simulink library "robot1"
PostLoadFcn:
  | robot1_BusGenerator
libraries: AtomicLibrary x3

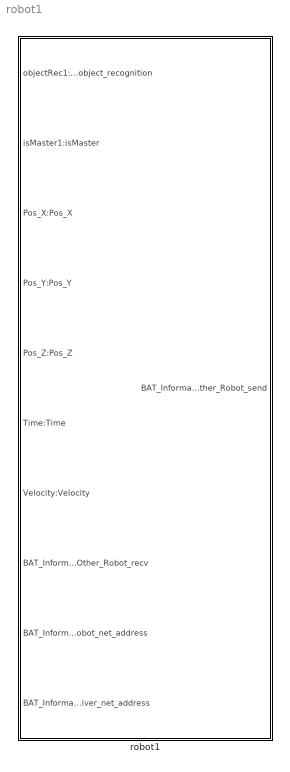
== system robot1 ==
  robot1 : Subsystem  Tag=id=_8vFAgJMGEeKkUdL0M2Clrg

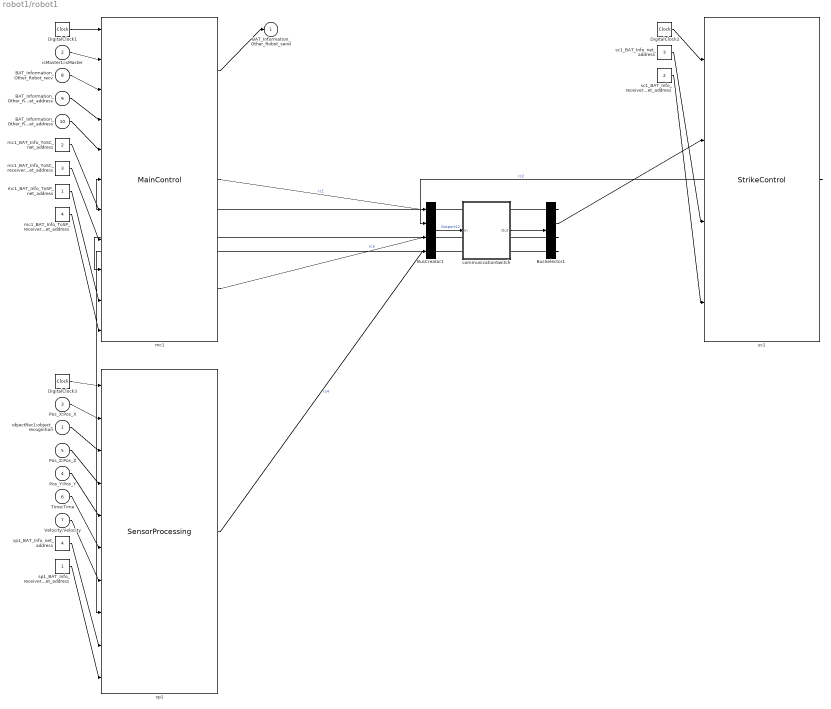
== system robot1/robot1 ==
  objectRec1:object_recognition : Inport  Tag=id=_98BUwJMGEeKkUdL0M2Clrg  Port=1  DataType=boolean  OutDataType=fixdt(1, 16)  OutScaling=2^0  OutDataTypeStr=boolean
  isMaster1:isMaster : Inport  Tag=id=_98QlUJMGEeKkUdL0M2Clrg  Port=2  DataType=boolean  OutDataType=fixdt(1, 16)  OutScaling=2^0  OutDataTypeStr=boolean
  Pos_X:Pos_X : Inport  Tag=id=_98nxsJMGEeKkUdL0M2Clrg  Port=3  DataType=boolean  OutDataType=fixdt(1, 16)  OutScaling=2^0  OutDataTypeStr=boolean
  Pos_Y:Pos_Y : Inport  Tag=id=_989v8JMGEeKkUdL0M2Clrg  Port=4  DataType=boolean  OutDataType=fixdt(1, 16)  OutScaling=2^0  OutDataTypeStr=boolean
  Pos_Z:Pos_Z : Inport  Tag=id=_99THIJMGEeKkUdL0M2Clrg  Port=5  DataType=boolean  OutDataType=fixdt(1, 16)  OutScaling=2^0  OutDataTypeStr=boolean
  Time:Time : Inport  Tag=id=_99svwJMGEeKkUdL0M2Clrg  Port=6  DataType=boolean  OutDataType=fixdt(1, 16)  OutScaling=2^0  OutDataTypeStr=boolean
  Velocity:Velocity : Inport  Tag=id=_9-QwcJMGEeKkUdL0M2Clrg  Port=7  DataType=boolean  OutDataType=fixdt(1, 16)  OutScaling=2^0  OutDataTypeStr=boolean
  BAT_Information_Other_Robot_recv : Inport  Tag=id=_9_CMgJMGEeKkUdL0M2Clrg  Port=8  DataType=auto  OutDataType=fixdt(1, 16)  OutScaling=2^0  UseBusObject=on  OutDataTypeStr=Inherit: auto
      settings: BusObject=PacketBus
  BAT_Information_Other_Robot_net_address : Inport  Tag=id=_9_CzkZMGEeKkUdL0M2Clrg  Port=9  DataType=uint8  OutDataType=fixdt(1, 16)  OutScaling=2^0  OutDataTypeStr=uint8
  BAT_Information_Other_Robot_receiver_net_address : Inport  Tag=id=_9_DaoJMGEeKkUdL0M2Clrg  Port=10  DataType=uint8  OutDataType=fixdt(1, 16)  OutScaling=2^0  OutDataTypeStr=uint8
  BAT_Information_Other_Robot_send : Outport  Tag=id=_9_CzkJMGEeKkUdL0M2Clrg  Port=1  DataType=auto  OutDataType=fixdt(1, 16)  OutScaling=2^0  UseBusObject=on  OutDataTypeStr=Inherit: auto
      settings: BusObject=PacketBus
  communicationSwitch : Subsystem  Tag=id=_8vJR8pMGEeKkUdL0M2Clrg
  BusCreator1 : BusCreator  Inputs=4  UseBusObject=on  Tag=id=_8vGOoJMGEeKkUdL0M2Clrg
      settings: BusObject=robot1_Bus
  BusSelector1 : BusSelector  OutputSignals=rc1,rc2,rc3,rc4  Tag=id=_8vGOoZMGEeKkUdL0M2Clrg
  mc1 : AtomicLibrary/MainControl  Tag=id=_8wMa0JMGEeKkUdL0M2Clrg
  DigitalClock1 : DigitalClock  Tag=id=_8wMa0ZMGEeKkUdL0M2Clrg  SampleTime=0.0010
  sc1 : AtomicLibrary/StrikeControl  Tag=id=_8wPeIZMGEeKkUdL0M2Clrg
  DigitalClock2 : DigitalClock  Tag=id=_8wQFMJMGEeKkUdL0M2Clrg  SampleTime=0.0010
  sp1 : AtomicLibrary/SensorProcessing  Tag=id=_8wShcZMGEeKkUdL0M2Clrg
  DigitalClock3 : DigitalClock  Tag=id=_8wTIgJMGEeKkUdL0M2Clrg  SampleTime=0.0010
  mc1_BAT_Info_ToSC_net_address : Constant  Tag=id=_94PA8ZMGEeKkUdL0M2Clrg  Value=2  OutDataTypeMode=uint8  OutDataTypeStr=uint8
  mc1_BAT_Info_ToSP_net_address : Constant  Tag=id=_94dDYZMGEeKkUdL0M2Clrg  Value=1  OutDataTypeMode=uint8  OutDataTypeStr=uint8
  sc1_BAT_Info_net_address : Constant  Tag=id=_94qewZMGEeKkUdL0M2Clrg  Value=3  OutDataTypeMode=uint8  OutDataTypeStr=uint8
  sp1_BAT_Info_net_address : Constant  Tag=id=_95kdsZMGEeKkUdL0M2Clrg  Value=4  OutDataTypeMode=uint8  OutDataTypeStr=uint8
  mc1_BAT_Info_ToSC_receiver_net_address : Constant  Tag=id=_GLOx5ZMHEeKkUdL0M2Clrg  Value=3  OutDataTypeMode=uint8  OutDataTypeStr=uint8
  sc1_BAT_Info_receiver_net_address : Constant  Tag=id=_GLQAAJMHEeKkUdL0M2Clrg  Value=2  OutDataTypeMode=uint8  OutDataTypeStr=uint8
  mc1_BAT_Info_ToSP_receiver_net_address : Constant  Tag=id=_GLZxBJMHEeKkUdL0M2Clrg  Value=4  OutDataTypeMode=uint8  OutDataTypeStr=uint8
  sp1_BAT_Info_receiver_net_address : Constant  Tag=id=_GLa_IZMHEeKkUdL0M2Clrg  Value=1  OutDataTypeMode=uint8  OutDataTypeStr=uint8
  wires:
  BusCreator1/1 -> communicationSwitch/1(In)  "Outport12"
  communicationSwitch/1(Out) -> BusSelector1/1
  DigitalClock1/1 -> mc1/1
  DigitalClock2/1 -> sc1/1
  DigitalClock3/1 -> sp1/1
  mc1_BAT_Info_ToSC_net_address/1 -> mc1/7
  mc1_BAT_Info_ToSP_net_address/1 -> mc1/10
  sc1_BAT_Info_net_address/1 -> sc1/3
  sp1_BAT_Info_net_address/1 -> sp1/9
  mc1/2 -> BusCreator1/1  "rc1"
  sc1/1 -> BusCreator1/2  "rc2"
  BusSelector1/2 -> sc1/2
  BusSelector1/1 -> mc1/6
  mc1_BAT_Info_ToSC_receiver_net_address/1 -> mc1/8
  sc1_BAT_Info_receiver_net_address/1 -> sc1/4
  mc1/3 -> BusCreator1/3  "rc3"
  sp1/1 -> BusCreator1/4  "rc4"
  BusSelector1/4 -> sp1/8
  BusSelector1/3 -> mc1/9
  mc1_BAT_Info_ToSP_receiver_net_address/1 -> mc1/11
  sp1_BAT_Info_receiver_net_address/1 -> sp1/10
  isMaster1:isMaster/1 -> mc1/2
  Pos_Z:Pos_Z/1 -> sp1/4
  Pos_Y:Pos_Y/1 -> sp1/5
  Pos_X:Pos_X/1 -> sp1/2
  Time:Time/1 -> sp1/6
  objectRec1:object_recognition/1 -> sp1/3
  Velocity:Velocity/1 -> sp1/7
  BAT_Information_Other_Robot_recv/1 -> mc1/3
  mc1/1 -> BAT_Information_Other_Robot_send/1
  BAT_Information_Other_Robot_receiver_net_address/1 -> mc1/5
  BAT_Information_Other_Robot_net_address/1 -> mc1/4

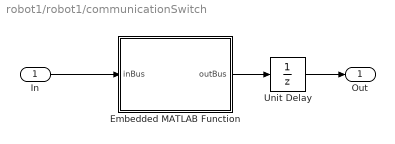
== system robot1/robot1/communicationSwitch ==
  In : Inport  Tag=id=_8vMVQJMGEeKkUdL0M2Clrg  Port=1  PortDimensions=-1  OutDataType=fixdt(1, 16)  OutScaling=2^0  UseBusObject=on
      settings: BusObject=robot1_Bus
  Out : Outport  Tag=id=_8vOKcJMGEeKkUdL0M2Clrg  Port=1  PortDimensions=-1  OutDataType=fixdt(1, 16)  OutScaling=2^0  UseBusObject=on
      settings: BusObject=robot1_Bus
  Unit Delay : UnitDelay  Tag=id=_8vPYkJMGEeKkUdL0M2Clrg  SampleTime=-1
  Embedded MATLAB Function : Stateflow chart  Tag=id=_8vPYkZMGEeKkUdL0M2Clrg
  wires:
  In/1 -> Embedded MATLAB Function/1(inBus)
  Unit Delay/1 -> Out/1
  Embedded MATLAB Function/1(outBus) -> Unit Delay/1

== matlab function robot1/communicationSwitch/Embedded MATLAB Function ==
  data: inBus input Bus: robot1_Bus; outBus output Bus: robot1_Bus
function outBus = BusImpl(inBus)
%#eml
eml.extrinsic('fieldnames','disp','setfield','fprintf');

busSize = 1;
queueSize = 10*busSize; %length of queue
numShuttles = 0; %Define data type
numShuttles = numel(fieldnames(inBus)); %Shuttles connected to the bus
assert(numShuttles <= 20) %Defines an upper bound for number of shuttles. 
%Important for static memory allocation. 
lookupTableSize = 200;



NOT_ASSIGNED = -1;

%We need persistent queues
persistent queue;
persistent lookupTable;

%Initialize the queues
if isempty(queue)
    queue = repmat(emptyPacket(), numShuttles, queueSize);
end

if isempty(lookupTable)
    lookupTable = repmat(NOT_ASSIGNED, lookupTableSize,1);
end

%Clean outbus
outBus = inBus;
for i = 1:numShuttles
    outBus = setfield(outBus, createRailCabName(i), emptyBus(busSize));
end

%Retrieve packets
for i = 1:numShuttles
    %Get current bus
    currentBus = getBusFromIndex(inBus, busSize, i);
    for j = 1:busSize
        %Read packet
        packet = getPacketFromBus(currentBus, j);
        
        %Check if new packet
        if isValid(packet, numShuttles)
             %Save sender bus element to lookup table
            if lookupTable(packet.from) == NOT_ASSIGNED
                lookupTable(packet.from) = i;
            end
            
            %Save packet in queue
            target = lookupTable(packet.to);
            %Destination unkown. Send to all unassigned.
            if target == NOT_ASSIGNED
                for k = 1:numShuttles
                    if(lookupTable(packet.from) ~= k)
                        queue(k,:) = enqueue(queue(k,:), packet); 
                    end
                end                
            %Destination known
            else 
                queue(target,:) = enqueue(queue(target,:), packet);
            end            
        end
    end

end

%Send packet from queue
for i = 1:numShuttles    
    currentBus = getBusFromIndex(outBus, busSize, i);
    for j = 1:busSize
        if ~isEmpty(queue(i,:))
            
            
            %Read last packet
            packet = front(queue(i,:));
            queue(i,:) = dequeue(queue(i,:)); 
            
%            if packet.msg ~= 255 %No ACK
%                fprintf('Sending on port %u[%u/%u]: %s', i, j, busSize, toString(packet));
%            end            
            
            %Save packet to bus
            currentBus = setPacketToBus(currentBus, j, packet);
            
        else
            break;
        end
    end 
    %Save bus
    outBus = setBusToIndex(outBus, i, currentBus);
end

%%%%%%%%%%%%%%%%%%%%%%%%%%%%%%%%%%%%%%%%%%%%%%%%%%%%%%%%%%%%%%%%%%%%%%%%%%%
%% BUS
%%%%%%%%%%%%%%%%%%%%%%%%%%%%%%%%%%%%%%%%%%%%%%%%%%%%%%%%%%%%%%%%%%%%%%%%%%%

function name = createRailCabName(index) %#eml
%Create name for the railcab used on the bus
eml.extrinsic('sprintf');
name = sprintf('rc%d', index);

function bus = getBusFromIndex(inBus, busSize, index) %eml
%Retrieve a PacketBus from the RailCaBbus
eml.extrinsic('getfield');
busName = createRailCabName(index);
bus = emptyBus(busSize);
bus = getfield(inBus, busName);

function rcBus = setBusToIndex(rcBus, index, packetBus) %eml
%Save a PacketBus to RailCabBus
eml.extrinsic('setfield');
busName = createRailCabName(index);
rcBus = setfield(rcBus, busName, packetBus);

function packet = getPacketFromBus(packetBus, index) %eml
%Retrieve a packet from the bus
packet = emptyPacket();
packet.from = packetBus.from(index);
packet.to = packetBus.to(index);
packet.msg = packetBus.msg(index);
packet.param = packetBus.param (index);
packet.pkgid = packetBus.pkgid(index);
packet.time = packetBus.time(index);

function packetBus = setPacketToBus(packetBus, index, packet) %eml
%Save a packet to the bus
packetBus.from(index) = packet.from;
packetBus.to(index) = packet.to;
packetBus.msg(index) = packet.msg;
packetBus.param (index) = packet.param;
packetBus.pkgid(index) = packet.pkgid;
packetBus.time(index) = packet.time;

function bus = emptyBus(size) %emp
%Create an empty bus
bus = struct('from', zeros(size,1,'uint8'),'to', zeros(size,1,'uint8'),'msg', zeros(size,1,'uint16'),'param', zeros(size,1,'double'),'pkgid', zeros(size,1,'uint32'), 'time', zeros(size,1,'double'));


%%%%%%%%%%%%%%%%%%%%%%%%%%%%%%%%%%%%%%%%%%%%%%%%%%%%%%%%%%%%%%%%%%%%%%%%%%%
%% PACKET
%%%%%%%%%%%%%%%%%%%%%%%%%%%%%%%%%%%%%%%%%%%%%%%%%%%%%%%%%%%%%%%%%%%%%%%%%%%
function packet = emptyPacket() %#eml
%Creates an empty packet
packet = struct('from', uint8(0),'to', uint8(0),'msg', uint16(0),'param', double(0.0),'pkgid', uint32(0), 'time', double(0));

function valid = isValid(packet, numShuttles) %#eml
%Checks wether the given packet is valid and transported by the bus
eml.extrinsic('getfield');
valid = false;
if packet.to > 0 && packet.to <= numShuttles 
    if packet.from > 0 && packet.from <= numShuttles
        valid = true;
    end
end

function packetString = toString(packet) %#eml
eml.extrinsic('sprintf');
packetString = sprintf('%3u: %u->%u :%3u (%.1f) @%.2f', packet.pkgid, packet.from, packet.to, packet.msg, packet.param, packet.time);

%%%%%%%%%%%%%%%%%%%%%%%%%%%%%%%%%%%%%%%%%%%%%%%%%%%%%%%%%%%%%%%%%%%%%%%%%%%
%% QUEUE
%%%%%%%%%%%%%%%%%%%%%%%%%%%%%%%%%%%%%%%%%%%%%%%%%%%%%%%%%%%%%%%%%%%%%%%%%%%

function queue = enqueue(queue, packet) %#eml
%Insert the packet at the end of the queue
eml.extrinsic('warning');
for i=1:length(queue)
    if queue(i).to == 0
        queue(i) = packet;
        return;
    end
end
%No empty entry found
warning('RailCab:Bus','Bus: buffer overflow for outgoing queue to %d', queue(1).to);

function queue = dequeue(queue) %#eml
%Removes the first packet of the queue
for i = 1:length(queue)-1
    queue(i) = queue(i+1);
    if queue(i).to == 0
        %end reached
        return;
    end
end
queue(length(queue)) = emptyPacket();

function packet = front(queue) %#eml
%Returns the first element from the queue
packet = queue(1);

function empty = isEmpty(queue) %#eml
%Checks whether the queue is empty or not
packet = queue(1);
if packet.to == 0
    empty = true;
else
    empty = false;
end
